simulink model "PendSim"  (R2019b)
settings: Solver=VariableStepAuto  StartTime=0.0  StopTime=30  RelTol=1e-3
InitFcn:
  | PendInit
values from neighbouring files (symbols this model uses):
  Ac = [(A-B*K)]    [PendInit.m]
  Bc = [B]    [PendInit.m]
  Cc = [C]    [PendInit.m]
  Dc = [D]    [PendInit.m]
  Kd = 1    [PendInit.m]
  Ki = 1    [PendInit.m]
  Kp = 100    [PendInit.m]
  Nbar = rscale(sys_ss,K)    [PendInit.m]    (also in rscale.m = Nu + K*Nx)
  P_cart_den = P_cart_den{1}    [PendInit.m]
  P_cart_num = P_cart_num{1}    [PendInit.m]
  P_pend_den = P_pend_den{1}    [PendInit.m]
  P_pend_num = P_pend_num{1}    [PendInit.m]
libraries: vrlib x3, simulink x1, sldrtlib x1
settings Model: Creator=STEVEN-USER  LastModifiedBy=STEVEN-USER

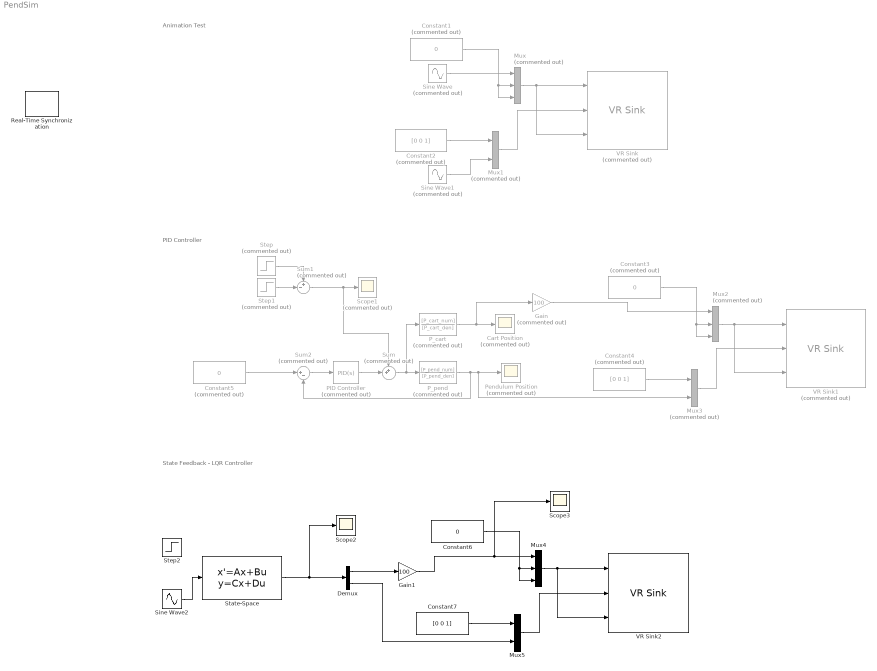
== system PendSim ==
  note: PID Controller
  note: State Feedback - LQR Controller
  note: Animation Test
  Cart Position : Scope  Commented=on
  Constant1 : Constant  Commented=on  Value=0
  Constant2 : Constant  Commented=on  Value=[0 0 1]
  Constant3 : Constant  Commented=on  Value=0
  Constant4 : Constant  Commented=on  Value=[0 0 1]
  Constant5 : Constant  Commented=on  Value=0
  Constant6 : Constant  Value=0
  Constant7 : Constant  Value=[0 0 1]
  Demux : Demux  Outputs=2
  Gain : Gain  Commented=on  Gain=100
  Gain1 : Gain  Gain=100
  Mux : Mux  Commented=on  Inputs=3
  Mux1 : Mux  Commented=on  Inputs=2
  Mux2 : Mux  Commented=on  Inputs=3
  Mux3 : Mux  Commented=on  Inputs=2
  Mux4 : Mux  Inputs=3
  Mux5 : Mux  Inputs=2
  PID Controller : simulink/Continuous/PID Controller  Commented=on  Controller=PID  Form=Parallel  TimeDomain=Continuous-time  SampleTime=-1  IntegratorMethod=Forward Euler  FilterMethod=Forward Euler  ControllerParametersSource=internal  P=Kp  I=Ki  D=Kd  UseFilter=on  N=100  TunerSelectOption=Transfer Function Based (PID Tuner App)  InitialConditionSource=internal  InitialConditionForIntegrator=0  InitialConditionForFilter=0  DifferentiatorICPrevScaledInput=0  ExternalReset=none  TrackingMode=off  Kt=1  LimitOutput=off  UpperSaturationLimit=inf  LowerSaturationLimit=-inf  LinearizeAsGain=on  AntiWindupMode=none  Kb=1  POutMin=[]  POutMax=[]  IOutMin=[]  IOutMax=[]  DOutMin=[]  DOutMax=[]  NOutMin=[]  NOutMax=[]  SumOutMin=[]  SumOutMax=[]  SaturationOutMin=[]  SaturationOutMax=[]  PParamMin=[]  PParamMax=[]  IParamMin=[]  IParamMax=[]  DParamMin=[]  DParamMax=[]  NParamMin=[]  NParamMax=[]  KbParamMin=[]  KbParamMax=[]  KtParamMin=[]  KtParamMax=[]  KbOutMin=[]  KbOutMax=[]  KtOutMin=[]  KtOutMax=[]  IntegratorOutMin=[]  IntegratorOutMax=[]  FilterOutMin=[]  FilterOutMax=[]  SumI1OutMin=[]  SumI1OutMax=[]  SumI2OutMin=[]  SumI2OutMax=[]  SumI3OutMin=[]  SumI3OutMax=[]  SumI4OutMin=[]  SumI4OutMax=[]  SumDOutMin=[]  SumDOutMax=[]  DifferentiatorOutMin=[]  DifferentiatorOutMax=[]  FilterDiffOutCoefMin=[]  FilterDiffOutCoefMax=[]  ReciprocalOutMin=[]  ReciprocalOutMax=[]  SumDenOutMin=[]  SumDenOutMax=[]  SumNumOutMin=[]  SumNumOutMax=[]  DivideOutMin=[]  DivideOutMax=[]  IntegratorContinuousStateAttributes=''  IntegratorStateMustResolveToSignalObject=off  IntegratorRTWStateStorageClass=Auto  FilterContinuousStateAttributes=''  FilterStateMustResolveToSignalObject=off  FilterRTWStateStorageClass=Auto  ParallelPVariant=InternalParameters  IdealPVariant=Disabled  IVariant=InternalParameters  DVariant=InternalParameters  IntegratorVariant=Continuous  SatVariant=Disabled  AWVariant=Passthrough  PCopyVariant=Disabled  TRVariant=Disabled  FdbkBlocksVariant=Forward  IdealPFdbkVariant=Disabled  SatFdbkVariant=Disabled  DerivativeFilterVariant=ContFilter  NVariant=InternalParameters  NCopyVariant=Disabled  FilterICVariant=InternalICsFilter  IntegratorICVariant=InternalICs  ExternalResetVariant=Disabled  TRSumVariant=Passthrough  SumFdbkVariant=Disabled  SumVariant=Sum_PID
  P_cart : TransferFcn  Commented=on  Numerator=[P_cart_num]  Denominator=[P_cart_den]
  P_pend : TransferFcn  Commented=on  Numerator=[P_pend_num]  Denominator=[P_pend_den]
  Pendulum Position : Scope  Commented=on
  Real-Time Synchronization : sldrtlib/Real-Time Synchronization  SampleTime=0.01  MaxMissedTicks=10  ShowMissedTicks=off  YieldWhenWaiting=off
  Scope1 : Scope  Commented=on
  Scope2 : Scope
  Scope3 : Scope
  Sine Wave : Sin  Commented=on  Amplitude=40  SampleTime=0
  Sine Wave1 : Sin  Commented=on  Amplitude=pi/2  SampleTime=0
  Sine Wave2 : Sin  Amplitude=.5  Frequency=2*pi  SampleTime=0
  State-Space : StateSpace  A=Ac  B=Bc*Nbar  C=Cc  D=Dc  InitialCondition=0
  Step : Step  Commented=on  After=20  SampleTime=0
  Step1 : Step  Commented=on  Time=1.1  After=20  SampleTime=0
  Step2 : Step  After=0.2  SampleTime=0
  Sum : Sum  Commented=on  Inputs=++|
  Sum1 : Sum  Commented=on  Inputs=+-|
  Sum2 : Sum  Commented=on  Inputs=|+-
  VR Sink : vrlib/VR Sink  Commented=on  InstantiateOnLoad=on  SampleTime=0.1  ViewEnable=on  RemoteChange=off  RemoteView=off  FieldsWritten=Plane_Square.translation.3.1.1.double#Plane_Square_0001.rotation.4.1.1.double#Plane_Square_0001.translation.3.1.1.double  WorldFileName=Pendulumn.wrl  AutoView=off  VideoDimensions=[]  AllowVariableSize=off
      settings: SourceProductName=Simulink
  VR Sink1 : vrlib/VR Sink  Commented=on  InstantiateOnLoad=on  SampleTime=0.1  ViewEnable=on  RemoteChange=off  RemoteView=off  FieldsWritten=Plane_Square.translation.3.1.1.double#Plane_Square_0001.rotation.4.1.1.double#Plane_Square_0001.translation.3.1.1.double  WorldFileName=Pendulumn.wrl  AutoView=off  VideoDimensions=[]  AllowVariableSize=off
      settings: SourceProductName=Simulink
  VR Sink2 : vrlib/VR Sink  InstantiateOnLoad=on  SampleTime=0.1  ViewEnable=on  RemoteChange=off  RemoteView=off  FieldsWritten=Plane_Square.translation.3.1.1.double#Plane_Square_0001.rotation.4.1.1.double#Plane_Square_0001.translation.3.1.1.double  WorldFileName=Pendulumn.wrl  AutoView=off  VideoDimensions=[]  AllowVariableSize=off
      settings: SourceProductName=Simulink
  wires:
  Sine Wave/1 -> Mux/1
  Constant1/1 -> Mux/3, Mux/2
  Mux/1 -> VR Sink/3, VR Sink/1
  Constant2/1 -> Mux1/1
  Sine Wave1/1 -> Mux1/2
  Mux1/1 -> VR Sink/2
  PID Controller/1 -> Sum/2
  Sum/1 -> P_cart/1, P_pend/1
  Sum2/1 -> PID Controller/1
  P_pend/1 -> Mux3/2, Pendulum Position/1, Sum2/2
  Constant5/1 -> Sum2/1
  Sum1/1 -> Sum/1, Scope1/1
  Mux2/1 -> VR Sink1/3, VR Sink1/1
  Mux3/1 -> VR Sink1/2
  Constant3/1 -> Mux2/3, Mux2/2
  Constant4/1 -> Mux3/1
  P_cart/1 -> Gain/1, Cart Position/1
  Gain/1 -> Mux2/1
  Step/1 -> Sum1/1
  Step1/1 -> Sum1/2
  State-Space/1 -> Demux/1, Scope2/1
  Constant7/1 -> Mux5/1
  Mux5/1 -> VR Sink2/2
  Mux4/1 -> VR Sink2/3, VR Sink2/1
  Demux/2 -> Mux5/2
  Constant6/1 -> Mux4/3, Mux4/2
  Sine Wave2/1 -> State-Space/1
  Gain1/1 -> Scope3/1, Mux4/1
  Demux/1 -> Gain1/1
